simulink model "modell_2"  (Simulink 7.8)
settings: Solver=ode45  StartTime=0.0  StopTime=10  MaxStep=1e-4  RelTol=1e-3
undefined symbols (not defined in the file or in its folder): dBW, Fs, get, Hz, sided, Two
libraries: dspstat3 x2, dspsnks4 x2, dsparch4 x1, simulink x1, dspspect3 x1, dspsigops x1
settings Model: Creator=svenhoffmann  LastModifiedBy=josef  ExtModeAutoUpdateStatusClock=off
settings OptimizationCC: InlineInvariantSignals=on  InitFltsAndDblsToZero=on
settings DebuggingCC: SaveWithParameterizedLinksMsg=none  SignalResolutionControl=TryResolveAllWithWarning  MultiTaskDSMMsg=warning  MultiTaskCondExecSysMsg=none  FcnCallInpInsideContextMsg=Use local settings  StrictBusMsg=None
settings RTWCC: IncludeERTFirstTime=on
settings GRTTargetCC: TargetFcnLib=ansi_tfl_tmw.mat

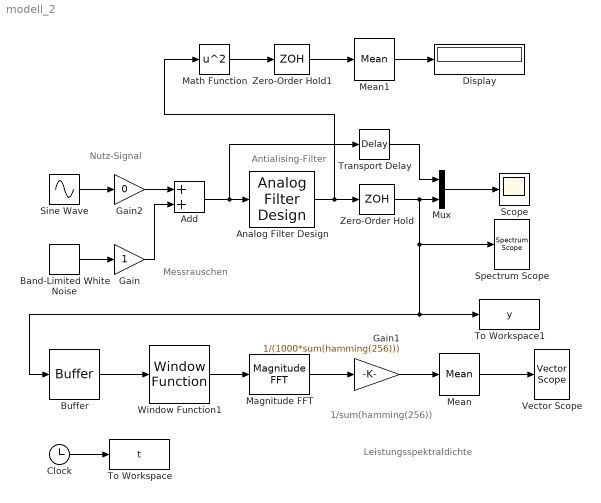
== system modell_2 ==
  note: Nutz-Signal
  note: Messrauschen
  note: Antialising-Filter
  note: Leistungsspektraldichte
  note: 1/sum(hamming(256))
  Add : Sum
  Analog Filter Design : dsparch4/Analog Filter Design  method=Butterworth  filttype=Lowpass  N=8  Wlo=2*pi*400  Whi=80  Rp=2  Rs=40
  Band-Limited White Noise : simulink/Sources/Band-Limited White Noise  Cov=[1/10000]  Ts=1/10000  seed=[23341]
  Buffer : Buffer  N=256
  Clock : Clock
  Display : Display
  Gain : Gain
  Gain1 : Gain  Gain=1/(1000*sum(hamming(256)))
  Gain2 : Gain  Gain=0
  Magnitude FFT : dspspect3/Magnitude FFT  mag_or_magsq=Magnitude squared  FFTImplementation=Auto  fftLenInherit=off  fftsize=256
  Math Function : Math  Operator=square  SaturateOnIntegerOverflow=on
  Mean : dspstat3/Mean  run=on  reset_popup=None  directionMode=Each column  dimension=1  treatSBRowAsCol=on  roiEnable=off  roiType=Rectangles  roiPortion=Entire ROI  roiOutput=Individual statistics for each ROI  roiFlag=off  outputDataTypeStr=Inherit: Same as accumulator  outputLastDataTypeStr=Inherit: Same as accumulator  outputMin=[]  outputMax=[]  roundingMode=Floor  overflowMode=off
  Mean1 : dspstat3/Mean  run=on  reset_popup=None  InputProcessing=Inherited (this choice will be removed - see release notes)  directionMode=Each column  dimension=1  treatSBRowAsCol=on  roiEnable=off  roiType=Rectangles  roiPortion=Entire ROI  roiOutput=Individual statistics for each ROI  roiFlag=off  outputDataTypeStr=Inherit: Same as accumulator  outputLastDataTypeStr=Inherit: Same as accumulator  outputMin=[]  outputMax=[]  roundingMode=Floor  overflowMode=off
  Mux : Mux  Inputs=2
  Scope : Scope
  Sine Wave : Sin  Frequency=2*pi*200  SampleTime=0
  Spectrum Scope : dspsnks4/Spectrum Scope  ScopeProperties=on  Domain=Frequency  HorizSpan=1  UseBuffer=on  BufferSize=256  Overlap=0  TreatMby1Signals=One channel  inpFftLenInherit=on  FFTlength=256  numAvg=30  DisplayProperties=off  AxisGrid=on  Memory=off  FrameNumber=on  AxisLegend=off  AxisZoom=off  OpenScopeAtSimStart=on  OpenScopeImmediately=off  FigPos=get(0,'defaultfigureposition')  AxisProperties=off  XUnits=Hertz  XRange=Two-sided ((-Fs/2...Fs/2])  XDisplay=0  InheritXIncr=on  XIncr=1.0  XLabel=Samples  XLimit=User-defined  YUnits=dBW/Hertz  XMax=500  XMin=-500  YLabel=dBW/Hz  LineProperties=off  wintypeSpecScope=Hamming  RsSpecScope=50  betaSpecScope=5  winsampSpecScope=Symmetric  XAxisParamsVer=6.9  isFrameUpgraded=on
      link override Periodogram: measurement=Mean-square spectrum  wintype=Hamming  winsamp=Symmetric  inheritFFT=off
      settings: YMin=-53.1298  YMax=-37.3837
  To Workspace : ToWorkspace  VariableName=t  SampleTime=-1  SaveFormat=Array
  To Workspace1 : ToWorkspace  VariableName=y  SampleTime=-1  SaveFormat=Array
  Transport Delay : TransportDelay  DelayTime=0.002
  Vector Scope : dspsnks4/Vector Scope  ScopeProperties=on  Domain=Frequency  HorizSpan=1  DisplayProperties=off  AxisGrid=on  Memory=off  FrameNumber=on  AxisLegend=off  AxisZoom=off  OpenScopeAtSimStart=on  OpenScopeImmediately=off  FigPos=get(0,'defaultfigureposition')  AxisProperties=off  XUnits=Hertz  XRange=[-Fs/2...Fs/2]  InheritXIncr=on  XIncr=1  XLabel=Time  XLimit=User-defined  XMin=-500  XMax=500  XStart=0  YUnits=dB  YLabel=dBW/Hz  LineProperties=off  XAxisParamsVer=6.8
      settings: YMin=-54.6702  YMax=-38.8438
  Window Function1 : dspsigops/Window Function  winmode=Apply window to input  wintype=Hamming  sampmode=Continuous  samptime=1  N=64  Rs=50  beta=10  winsamp=Symmetric  UserWindow=hamming  OptParams=off  UserParams={'symmetric'}  RowConvenienceOn=on  dataType=double  isSigned=on  wordLen=16  udDataType=sfix(16)  fracBitsMode=Best precision  numFracBits=15  roundingMode=Floor  overflowMode=off  numSidelobes=4  sidelobeLevel=-30
  Zero-Order Hold : ZeroOrderHold  SampleTime=1/1000
  Zero-Order Hold1 : ZeroOrderHold  SampleTime=1/5000
  wires:
  Band-Limited White Noise/1 -> Gain/1
  Sine Wave/1 -> Gain2/1
  Gain/1 -> Add/2
  Add/1 -> Analog Filter Design/1, Transport Delay/1
  Analog Filter Design/1 -> Zero-Order Hold/1, Math Function/1
  Zero-Order Hold/1 -> Mux/2, Spectrum Scope/1, Buffer/1, To Workspace1/1
  Transport Delay/1 -> Mux/1
  Mux/1 -> Scope/1
  Buffer/1 -> Window Function1/1
  Magnitude FFT/1 -> Gain1/1
  Mean/1 -> Vector Scope/1
  Gain1/1 -> Mean/1
  Math Function/1 -> Zero-Order Hold1/1
  Mean1/1 -> Display/1
  Zero-Order Hold1/1 -> Mean1/1
  Gain2/1 -> Add/1
  Clock/1 -> To Workspace/1
  Window Function1/1 -> Magnitude FFT/1
